simulink model "B_values"  (R2020a)
settings: Solver=VariableStepAuto  StartTime=0.0  StopTime=10.0  RelTol=1e-3
settings Model: Creator=emami  LastModifiedBy=emami

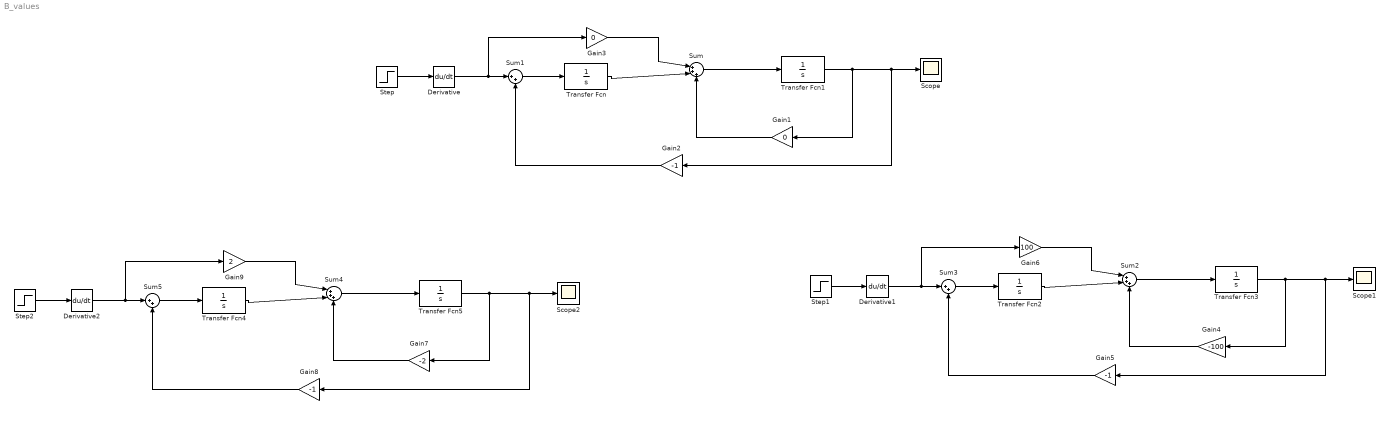
== system B_values ==
  Derivative : Derivative
  Derivative1 : Derivative
  Derivative2 : Derivative
  Gain1 : Gain  Gain=0
  Gain2 : Gain  Gain=-1
  Gain3 : Gain  Gain=0
  Gain4 : Gain  Gain=-100
  Gain5 : Gain  Gain=-1
  Gain6 : Gain  Gain=100
  Gain7 : Gain  Gain=-2
  Gain8 : Gain  Gain=-1
  Gain9 : Gain  Gain=2
  Scope : Scope
  Scope1 : Scope
  Scope2 : Scope
  Step : Step  Time=0.001  After=10  SampleTime=0
  Step1 : Step  Time=0.001  After=10  SampleTime=0
  Step2 : Step  Time=0.001  After=10  SampleTime=0
  Sum : Sum  Inputs=|+++
  Sum1 : Sum  Inputs=|++
  Sum2 : Sum  Inputs=|+++
  Sum3 : Sum  Inputs=|++
  Sum4 : Sum  Inputs=|+++
  Sum5 : Sum  Inputs=|++
  Transfer Fcn{,1..5} (6 alike) : TransferFcn  Denominator=[1 0]
  wires:
  Gain2/1 -> Sum1/2
  Sum1/1 -> Transfer Fcn/1
  Transfer Fcn/1 -> Sum/2
  Gain1/1 -> Sum/3
  Transfer Fcn1/1 -> Gain1/1, Gain2/1, Scope/1
  Gain3/1 -> Sum/1
  Sum/1 -> Transfer Fcn1/1
  Step/1 -> Derivative/1
  Derivative/1 -> Gain3/1, Sum1/1
  Gain6/1 -> Sum2/1
  Step1/1 -> Derivative1/1
  Gain4/1 -> Sum2/3
  Transfer Fcn2/1 -> Sum2/2
  Sum2/1 -> Transfer Fcn3/1
  Sum3/1 -> Transfer Fcn2/1
  Transfer Fcn3/1 -> Gain4/1, Gain5/1, Scope1/1
  Gain5/1 -> Sum3/2
  Derivative1/1 -> Gain6/1, Sum3/1
  Sum5/1 -> Transfer Fcn4/1
  Transfer Fcn5/1 -> Gain7/1, Gain8/1, Scope2/1
  Gain8/1 -> Sum5/2
  Gain9/1 -> Sum4/1
  Sum4/1 -> Transfer Fcn5/1
  Transfer Fcn4/1 -> Sum4/2
  Gain7/1 -> Sum4/3
  Derivative2/1 -> Gain9/1, Sum5/1
  Step2/1 -> Derivative2/1
